simulink model "Gbx_Data"  (R2016b)
settings: configuration reference "CodeGenConfigSet" (kept outside this file)
values from neighbouring files (symbols this model uses):
  Gbx_nIdlDes_C = Calibration.Parameter    [init_Gbx_Data.m]
  Gbx_rFanClgDem_C = Calibration.Parameter    [init_Gbx_Data.m]
  Gbx_rTrq_C = Calibration.Parameter    [init_Gbx_Data.m]
  Gbx_stOvrSpdDem_C = Calibration.Parameter    [init_Gbx_Data.m]
  Gbx_tClntDes_C = Calibration.Parameter    [init_Gbx_Data.m]
settings Model: Creator=lenovo  LastModifiedBy=bianxuyin
settings ConfigSetRef: SourceLocation=Base Workspace

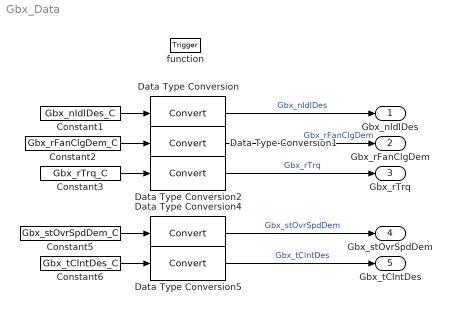
== system Gbx_Data ==
  function : TriggerPort  TriggerType=function-call  VariantControl=Variant
  Constant1 : Constant  Value=Gbx_nIdlDes_C
  Constant2 : Constant  Value=Gbx_rFanClgDem_C
  Constant3 : Constant  Value=Gbx_rTrq_C
  Constant5 : Constant  Value=Gbx_stOvrSpdDem_C
  Constant6 : Constant  Value=Gbx_tClntDes_C
  Data Type Conversion{,1..2,4..5} (5 alike) : DataTypeConversion
  Gbx_nIdlDes : Outport  Tag=rpm  Description=Desired idle speed setpoint for AT gear box rpm  OutMin=-6000  OutMax=6000  OutDataTypeStr=EngSpeed_rpm
  Gbx_rFanClgDem : Outport  Tag=%  Description=Percentage of fan cooling demand  Port=2  OutMin=-300  OutMax=300  OutDataTypeStr=Prc_100_rate
  Gbx_rTrq : Outport  Description=Transmission function information from Gearbox ECU(including Torque converter)  Port=3  OutMin=-100  OutMax=100  OutDataTypeStr=TransRatio
  Gbx_stOvrSpdDem : Outport  Description=status of engine overspeed request  Port=4  OutMin=0  OutMax=255  OutDataTypeStr=State_uint8
  Gbx_tClntDes : Outport  Tag=deg  Description=Setpoint value of the coolant temperature (via CAN)  Port=5  OutMin=-150  OutMax=150  OutDataTypeStr=Temp_deg
  wires:
  Constant1/1 -> Data Type Conversion/1
  Constant2/1 -> Data Type Conversion1/1
  Constant3/1 -> Data Type Conversion2/1
  Constant5/1 -> Data Type Conversion4/1
  Constant6/1 -> Data Type Conversion5/1
  Data Type Conversion/1 -> Gbx_nIdlDes/1  "Gbx_nIdlDes"
  Data Type Conversion1/1 -> Gbx_rFanClgDem/1  "Gbx_rFanClgDem"
  Data Type Conversion2/1 -> Gbx_rTrq/1  "Gbx_rTrq"
  Data Type Conversion4/1 -> Gbx_stOvrSpdDem/1  "Gbx_stOvrSpdDem"
  Data Type Conversion5/1 -> Gbx_tClntDes/1  "Gbx_tClntDes"
